simulink model "week2"  (R2018b)
settings: Solver=VariableStepAuto  StartTime=0.0  StopTime=10  RelTol=1e-3
settings Model: Creator=天霸动霸tua  LastModifiedBy=天霸动霸tua

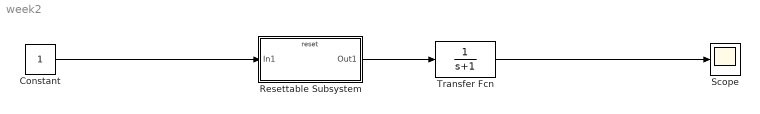
== system week2 ==
  Constant : Constant
  Resettable Subsystem : Subsystem  TreatAsAtomicUnit=on
      mask Display: disp('PID控制器')
  Scope : Scope
  Transfer Fcn : TransferFcn  Denominator=[1 1]
  wires:
  Constant/1 -> Resettable Subsystem/1(In1)
  Resettable Subsystem/1(Out1) -> Transfer Fcn/1
  Transfer Fcn/1 -> Scope/1

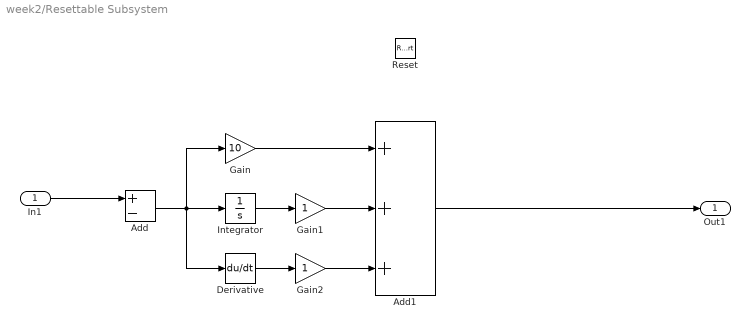
== system week2/Resettable Subsystem ==
  In1 : Inport
  Reset : ResetPort  DisableCoverage=on
  Add : Sum  Inputs=+-
  Add1 : Sum  Inputs=+++
  Derivative : Derivative
  Gain : Gain  Gain=10
  Gain1 : Gain
  Gain2 : Gain
  Integrator : Integrator
  Out1 : Outport
  wires:
  In1/1 -> Add/1
  Add/1 -> Derivative/1, Integrator/1, Gain/1
  Derivative/1 -> Gain2/1
  Gain/1 -> Add1/1
  Integrator/1 -> Gain1/1
  Gain2/1 -> Add1/3
  Gain1/1 -> Add1/2
  Add1/1 -> Out1/1
